simulink model "CC_CarExample_template"  (R2022b)
settings: Solver=VariableStepAuto  StartTime=0.0  StopTime=10.0  RelTol=1e-3
settings Model: Creator=sprinkle  LastModifiedBy=sprinkle
settings SolverCC: AlgebraicLoopSolver=TrustRegion
settings DebuggingCC: UnconnectedInputMsg=warning  UnconnectedOutputMsg=warning  UnconnectedLineMsg=warning  SFMachineParentedDataDiag=warning
settings ModelReferenceCC: EnableRefExpFcnMdlSchedulingChecks=on

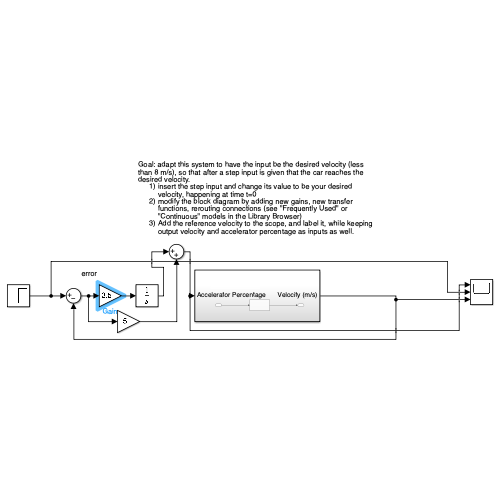
[thumbnail: Simulink's stored preview of the top-level diagram]
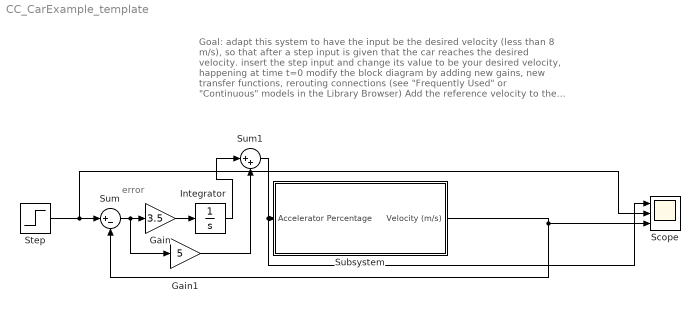
== system CC_CarExample_template ==
  note: error
  note: Goal: adapt this system to have the input be the desired velocity (less than 8 m/s), so that after a step input is given that the car reaches the desired velocity.
      | insert the step input and change its value to be your desired velocity, happening at time t=0
      | modify the block diagram by adding new gains, new transfer functions, rerouting connections (see "Frequently Used" or "Continuous" models in the Library Browser)
      | Add the reference velocity to the scope, and label it, while keeping output velocity and accelerator percentage as inputs as well.
  Gain : Gain  Gain=3.5
  Gain1 : Gain  Gain=5
  Integrator : Integrator
  Scope : Scope  NumInputPorts=3
  Step : Step  After=8  SampleTime=0
  Subsystem : Subsystem
  Sum : Sum  Inputs=|+-
  Sum1 : Sum  Inputs=|++
  wires:
  Subsystem/1(Velocity (m/s)) -> Scope/3, Sum/2
  Step/1 -> Scope/2, Sum/1
  Sum/1 -> Gain1/1, Gain/1
  Gain/1 -> Integrator/1
  Integrator/1 -> Sum1/1
  Sum1/1 -> Scope/1, Subsystem/1(Accelerator Percentage)
  Gain1/1 -> Sum1/2

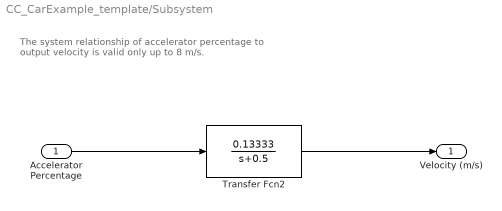
== system CC_CarExample_template/Subsystem ==
  note: The system relationship of accelerator percentage to output velocity is valid only up to 8 m/s.
  Accelerator Percentage : Inport
  Transfer Fcn2 : TransferFcn  Numerator=[0.13333]  Denominator=[1 0.5]
  Velocity (m/s) : Outport
  wires:
  Accelerator Percentage/1 -> Transfer Fcn2/1
  Transfer Fcn2/1 -> Velocity (m/s)/1
